simulink model "vibrations_pitch_v1"  (R2018b)
settings: Solver=VariableStepAuto  StartTime=0.0  StopTime=25  FixedStep=1e-4  MaxStep=1e-4  RelTol=1e-10
PreLoadFcn:
  | track_gen;
  | parameters_pitch;
InitFcn:
  | parameters_pitch;
  | track_gen;
values from neighbouring files (symbols this model uses):
  c = [0 l2*c2-l1*c1 k2*l2-k1*l1]    [analytical_soln.m]    (also in parameters_pitch.m = 100)
  Iyy = 115    [parameters_pitch.m]
  k = 7000    [parameters_pitch.m]
  L_back = 0.63    [parameters_pitch.m]
  L_front = 0.62    [parameters_pitch.m]
  m_pod = 300    [analytical_soln.m]    (also in parameters_pitch.m)
  m_wheel = 0.25    [parameters_pitch.m]
settings Model: Creator=Arturas  LastModifiedBy=dcarb
settings DebuggingCC: LibraryContextMissingDiagnostic=none
settings SFSimCC: SimUseLocalCustomCode=off
settings RTWCC: RTWUseLocalCustomCode=off

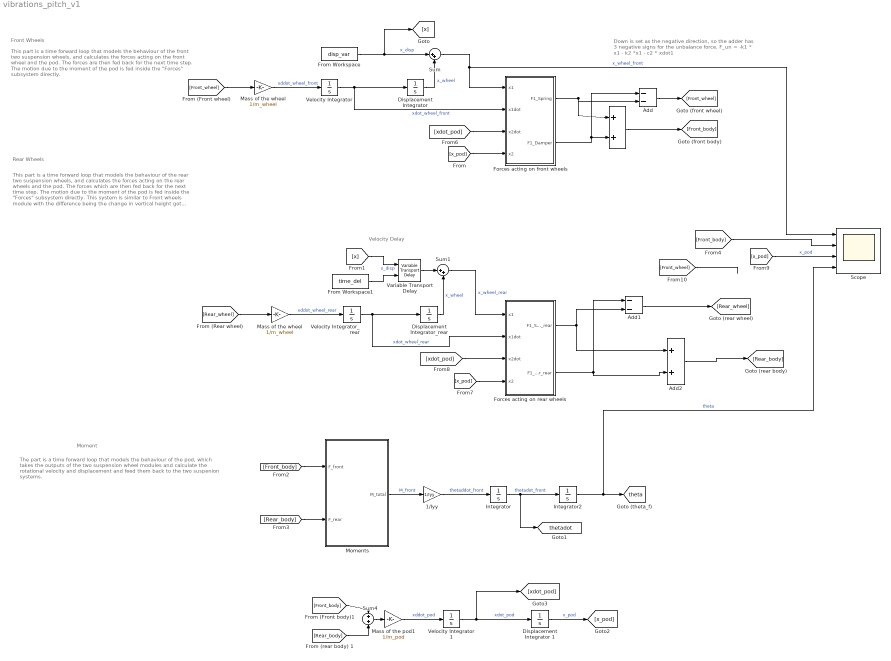
== system vibrations_pitch_v1 ==
  note: Rear Wheels
  note: Front Wheels
  note: Down is set as the negative direction, so the
      | adder has 3 negative signs for the unbalance force.
      | F_un = -k1 * x1 - k2 *x1 - c2 * xdot1
  note: This part is a time forward loop that models the behaviour of
      | the front two suspension wheels, and calculates the forces acting on the front wheel and the pod. The forces are then fed back for the next time step.
      |
      | The motion due to the moment of the pod is fed inside the "Forces" subsystem directly.
  note: Moment
  note: This part is a time forward loop that models the behaviour of
      | the rear two suspension wheels, and calculates the forces acting on
      | the rear wheels and the pod. The forces which are then fed back for the next time step.
      |
      | The motion due to the moment of the pod is fed inside the "Forces" subsystem directly.
      |
      | This system is similar to Front wheels module with the difference being the change in vertical height got delayed by:
      | time = translational velocity / horizontal displacement between the front and rear wheels
  note: The part is a time forward loop that models the behaviour of
      | the pod, which takes the outputs of the two suspension wheel modules and
      | calculate the rotational velocity and displacement and feed
      | them back to the two suspenion systems.
  note: Velocity Delay
  " " : Sum
  1/Iyy : Gain  Gain=1/Iyy
  Add : Sum  Inputs=--
  Add1 : Sum  Inputs=--
  Add2 : Sum
  Displacement Integrator : Integrator
  Displacement Integrator 1 : Integrator
  "Displacement Integrator_rear " : Integrator
  Forces acting on front wheels : Subsystem
  Forces acting on rear wheels : Subsystem
  From Workspace : FromWorkspace  VariableName=disp_var  Interpolate=off  OutputAfterFinalValue=Holding final value
  From Workspace1 : FromWorkspace  VariableName=time_del
  Integrator : Integrator
  Integrator2 : Integrator
  Mass of the pod1 : Gain  Gain=1/m_pod
  Mass of the wheel : Gain  Gain=1/m_wheel
  "Mass of the wheel " : Gain  Gain=1/m_wheel
  Moments : Subsystem
  Scope : Scope  NumInputPorts=4
  Sum : Sum  Inputs=|++
  Sum1 : Sum  Inputs=|++
  Sum4 : Sum
  Variable Transport Delay : VariableTransportDelay  MaximumDelay=10  TransDelayFeedthrough=on
  Velocity Integrator : Integrator
  Velocity Integrator 1 : Integrator
  Velocity Integrator_rear : Integrator
  tag scope: theta=global, thetadot=global
  wires:
  Moments/1(M_total) -> 1/Iyy/1  "M_front"
  Integrator2/1 -> [theta], Scope/4  "theta"
  [Front_body] -> Moments/1(F_front)
  [Rear_body] -> Moments/2(F_rear)
  Mass of the wheel/1 -> Velocity Integrator/1  "xddot_wheel_front"
  "Displacement Integrator_rear "/1 -> Sum1/2  "x_wheel"
  [Rear_wheel] -> "Mass of the wheel "/1
  Velocity Integrator_rear/1 -> Forces acting on rear wheels/2(x1dot), "Displacement Integrator_rear "/1  "xdot_wheel_rear"
  Add1/1 -> [Rear_wheel]
  Sum1/1 -> Forces acting on rear wheels/1(x1)  "x_wheel_rear"
  [Front_wheel] -> Mass of the wheel/1
  Sum/1 -> Forces acting on front wheels/1(x1), Scope/1  "x_wheel_front"
  Velocity Integrator/1 -> Forces acting on front wheels/2(x1dot), Displacement Integrator/1  "xdot_wheel_front"
  Displacement Integrator/1 -> Sum/2  "x_wheel"
  "Mass of the wheel "/1 -> Velocity Integrator_rear/1  "xddot_wheel_rear"
  Integrator/1 -> [thetadot], Integrator2/1  "thetadot_front"
  Forces acting on front wheels/1(F1_Spring) -> Add/2, " "/1
  1/Iyy/1 -> Integrator/1  "thetaddot_front"
  Forces acting on rear wheels/1(F1_Spring_rear) -> Add1/2, Add2/1
  Variable Transport Delay/1 -> Sum1/1
  " "/1 -> [Front_body]
  Forces acting on front wheels/2(F1_Damper) -> Add/1, " "/2
  Forces acting on rear wheels/2(F1_Damper_rear) -> Add2/2, Add1/1
  Add2/1 -> [Rear_body]
  Mass of the pod1/1 -> Velocity Integrator 1/1  "xddot_pod"
  Velocity Integrator 1/1 -> [xdot_pod], Displacement Integrator 1/1  "xdot_pod"
  [Front_body] -> Sum4/1
  Sum4/1 -> Mass of the pod1/1
  [Rear_body] -> Sum4/2
  Displacement Integrator 1/1 -> [x_pod]  "x_pod"
  [x_pod] -> Forces acting on front wheels/4(x2)
  [xdot_pod] -> Forces acting on front wheels/3(x2dot)
  [xdot_pod] -> Forces acting on rear wheels/3(x2dot)
  [x_pod] -> Forces acting on rear wheels/4(x2)
  [x] -> Variable Transport Delay/1  "x_disp"
  [x_pod] -> Scope/3  "x_pod"
  From Workspace/1 -> [x], Sum/1  "x_disp"
  [Front_wheel] -> ?
  From Workspace1/1 -> Variable Transport Delay/2
  [Front_body] -> Scope/2
  ? -> ?
  Add/1 -> [Front_wheel]

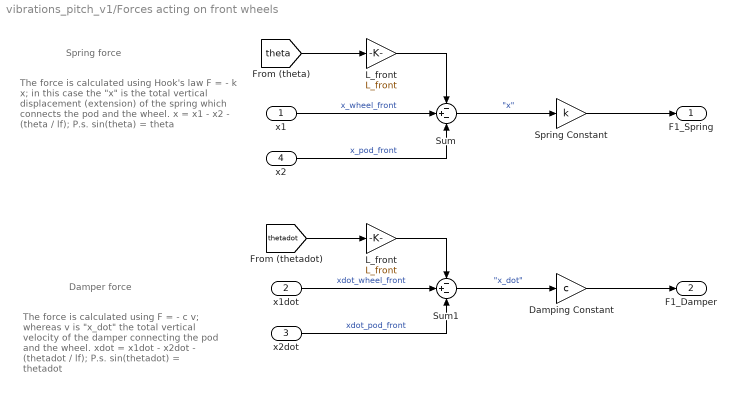
== system vibrations_pitch_v1/Forces acting on front wheels ==
  note: Spring force
  note: The force is calculated using Hook's law
      | F = - k x; in this case the "x" is the total
      | vertical displacement (extension) of the
      | spring which connects the pod and the wheel.
      | x = x1 - x2 - (theta / lf);
      | P.s. sin(theta) = theta
  note: Damper force
  note: The force is calculated using F = - c v;
      | whereas v is "x_dot" the total vertical
      | velocity of the damper connecting
      | the pod and the wheel.
      | xdot = x1dot - x2dot - (thetadot / lf);
      | P.s. sin(thetadot) = thetadot
  x1 : Inport
  x1dot : Inport  Port=2
  x2dot : Inport  Port=3
  x2 : Inport  Port=4
  Damping Constant : Gain  Gain=c
  L_front : Gain  Gain=L_front
  "L_front " : Gain  Gain=L_front
  Spring Constant : Gain  Gain=k
  Sum : Sum  Inputs=-+-
  Sum1 : Sum  Inputs=-+-
  F1_Spring : Outport
  F1_Damper : Outport  Port=2
  wires:
  x1/1 -> Sum/2  "x_wheel_front"
  x2/1 -> Sum/3  "x_pod_front"
  Sum/1 -> Spring Constant/1  "\"x\""
  Spring Constant/1 -> F1_Spring/1
  x1dot/1 -> Sum1/2  "xdot_wheel_front"
  x2dot/1 -> Sum1/3  "xdot_pod_front"
  Sum1/1 -> Damping Constant/1  "\"x_dot\""
  Damping Constant/1 -> F1_Damper/1
  [thetadot] -> "L_front "/1
  "L_front "/1 -> Sum1/1
  L_front/1 -> Sum/1
  [theta] -> L_front/1

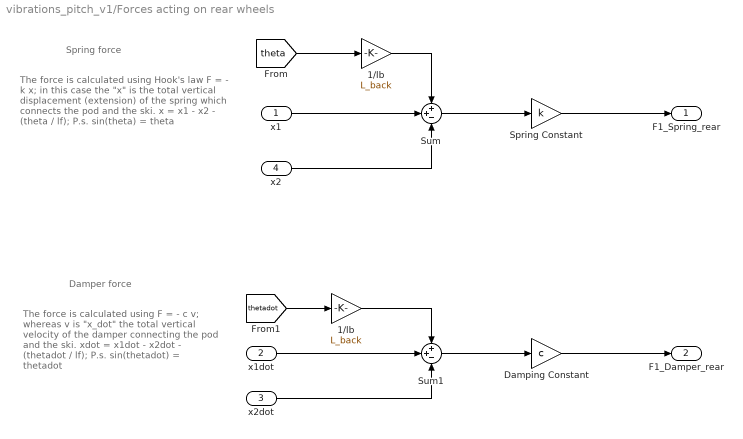
== system vibrations_pitch_v1/Forces acting on rear wheels ==
  note: Spring force
  note: The force is calculated using Hook's law
      | F = - k x; in this case the "x" is the total
      | vertical displacement (extension) of the
      | spring which connects the pod and the ski.
      | x = x1 - x2 - (theta / lf);
      | P.s. sin(theta) = theta
  note: Damper force
  note: The force is calculated using F = - c v;
      | whereas v is "x_dot" the total vertical
      | velocity of the damper connecting
      | the pod and the ski.
      | xdot = x1dot - x2dot - (thetadot / lf);
      | P.s. sin(thetadot) = thetadot
  x1 : Inport
  x1dot : Inport  Port=2
  x2dot : Inport  Port=3
  x2 : Inport  Port=4
  1/lb : Gain  Gain=L_back
  "1/lb " : Gain  Gain=L_back
  Damping Constant : Gain  Gain=c
  Spring Constant : Gain  Gain=k
  Sum : Sum  Inputs=++-
  Sum1 : Sum  Inputs=++-
  F1_Spring_rear : Outport
  F1_Damper_rear : Outport  Port=2
  wires:
  x1/1 -> Sum/2
  x2/1 -> Sum/3
  Sum/1 -> Spring Constant/1
  Spring Constant/1 -> F1_Spring_rear/1
  x1dot/1 -> Sum1/2
  x2dot/1 -> Sum1/3
  Sum1/1 -> Damping Constant/1
  Damping Constant/1 -> F1_Damper_rear/1
  [theta] -> 1/lb/1
  [thetadot] -> "1/lb "/1
  "1/lb "/1 -> Sum1/1
  1/lb/1 -> Sum/1

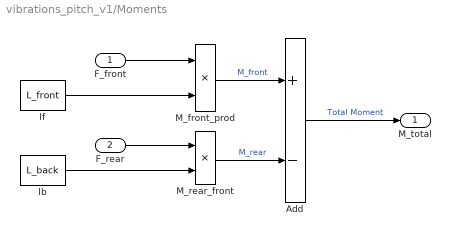
== system vibrations_pitch_v1/Moments ==
  F_front : Inport
  F_rear : Inport  Port=2
  Add : Sum  Inputs=+-
  M_front_prod : Product
  M_rear_front : Product
  lb : Constant  Value=L_back
  lf : Constant  Value=L_front
  M_total : Outport
  wires:
  F_front/1 -> M_front_prod/1
  lf/1 -> M_front_prod/2
  M_front_prod/1 -> Add/1  "M_front"
  lb/1 -> M_rear_front/2
  F_rear/1 -> M_rear_front/1
  M_rear_front/1 -> Add/2  "M_rear"
  Add/1 -> M_total/1  "Total Moment"
